simulink model "HVDCMMCInterconnection"  (R2023b)
settings: Solver=FixedStepDiscrete  StartTime=0.0  StopTime=10  FixedStep=Ts_Power  RelTol=1e-4
PreLoadFcn:
  | HVDCMMCInterconnectionParam
StartFcn:
  | tic
StopFcn:
  | toc
values from neighbouring files (symbols this model uses):
  C_PM = 1.758e-3    (= 0.001758)    [HVDCMMCInterconnectionParam.m]
  Cg = 50e-9    (= 5e-08)    [HVDCMMCInterconnectionParam.m]
  D_R = 0.001    [HVDCMMCInterconnectionParam.m]
  D_Rs = 1e8    (= 100000000)    [HVDCMMCInterconnectionParam.m]
  D_Vf = 0    [HVDCMMCInterconnectionParam.m]
  Fnom = 50    [HVDCMMCInterconnectionParam.m]
  HRM = 2    [HVDCMMCInterconnectionParam.m]
  Ki_Ireg = 6    [HVDCMMCInterconnectionParam.m]
  Ki_Preg = 1.0    (= 1)    [HVDCMMCInterconnectionParam.m]
  Ki_Qreg = 1.0    (= 1)    [HVDCMMCInterconnectionParam.m]
  Ki_VDCreg = 100    [HVDCMMCInterconnectionParam.m]
  Kp_Ireg = 0.6    [HVDCMMCInterconnectionParam.m]
  Kp_Preg = 0.5/3    (= 0.166666666667)    [HVDCMMCInterconnectionParam.m]
  Kp_Qreg = 0.5/3    (= 0.166666666667)    [HVDCMMCInterconnectionParam.m]
  Kp_VDCreg = 4    [HVDCMMCInterconnectionParam.m]
  L_cable = 15e-3    (= 0.015)    [HVDCMMCInterconnectionParam.m]
  Larm = Larm_pu*(Zb_ac/(2*pi*Fnom))    [HVDCMMCInterconnectionParam.m]
  Lff = Larm_pu/2    (= 0.075)    [HVDCMMCInterconnectionParam.m]
  Limits_Ireg = [ 2.0  -2.0]    [HVDCMMCInterconnectionParam.m]
  Limits_Preg = [ 1.2, 0.8 ]    [HVDCMMCInterconnectionParam.m]
  Limits_Qreg = [ 0.25, -0.25 ]    [HVDCMMCInterconnectionParam.m]
  Limits_VDCreg = [ 2.0  -2.0]    [HVDCMMCInterconnectionParam.m]
  Lxfo = 0.12    [HVDCMMCInterconnectionParam.m]
  Nb_PM = 36    [HVDCMMCInterconnectionParam.m]
  Pnom = 1000e6    (= 1000000000)    [HVDCMMCInterconnectionParam.m]
  R_cable = 0.5    [HVDCMMCInterconnectionParam.m]
  R_startup = 400    [HVDCMMCInterconnectionParam.m]
  Rarm = Rarm_pu*Zb_ac    [HVDCMMCInterconnectionParam.m]
  Rff = Rarm_pu/2    (= 0.00075)    [HVDCMMCInterconnectionParam.m]
  Rg = 100    [HVDCMMCInterconnectionParam.m]
  Rxfo = 0.003    [HVDCMMCInterconnectionParam.m]
  Slope_Pref = 0.5    [HVDCMMCInterconnectionParam.m]
  Slope_Qref = 0.5    [HVDCMMCInterconnectionParam.m]
  Slope_Vdc_ref = Vnom_dc/5    (= 128000)    [HVDCMMCInterconnectionParam.m]
  Tbrk1_On = 0.1    [HVDCMMCInterconnectionParam.m]
  Tbrk2_On = 1.0    (= 1)    [HVDCMMCInterconnectionParam.m]
  Tdeblock = 1.5    [HVDCMMCInterconnectionParam.m]
  Tfault = 9999    [HVDCMMCInterconnectionParam.m]
  Ton_Converter2 = 4    [HVDCMMCInterconnectionParam.m]
  Ton_PQreg = 4    [HVDCMMCInterconnectionParam.m]
  Ton_VDCreg = 1.5    [HVDCMMCInterconnectionParam.m]
  Ts = Ts_Control    (= 4e-05)    [HVDCMMCInterconnectionParam.m]    (also in power_circ2ss_sps_calc.m = 1e-06)
  Ts_Control = 40e-6    (= 4e-05)    [HVDCMMCInterconnectionParam.m]
  Ts_Power = 20e-6    (= 2e-05)    [HVDCMMCInterconnectionParam.m]
  Vb_ac = sqrt(2/3)*Vnom_sec    [HVDCMMCInterconnectionParam.m]
  Vb_dc = Vnom_dc    (= 640000)    [HVDCMMCInterconnectionParam.m]
  Vc0_PM = 0    [HVDCMMCInterconnectionParam.m]
  Vnom_dc = 640e3    (= 640000)    [HVDCMMCInterconnectionParam.m]
  Vnom_prim = 400e3    (= 400000)    [HVDCMMCInterconnectionParam.m]
  Vnom_sec = 333e3    (= 333000)    [HVDCMMCInterconnectionParam.m]
  w = 2*pi*Fnom    (= 314.159265359)    [HVDCMMCInterconnectionParam.m]
undefined symbols (not defined in the file or in its folder): ACDC, ACDC3, DiscIntNeverNeededParam, gcbh, Pcc, S, sps_AC, sps_rtmsupport
libraries: simulink x61, spsControlledVoltageSourceLib x56, spsCurrentMeasurementLib x56, spsDiodeLib x40, spsSeriesRLCBranchLib x32, spsVoltageMeasurementLib x20, powerlib_extras x9, spsHalfBridgeMMCmodel x8, spsGroundLib x7, spsSecondOrderFilterLib x6, spsabctodq0Lib x6, spsMeanLib x3
(part 2 of 11)

== system HVDCMMCInterconnection/3ph SM1 ==
  Uref_An : Inport
  An_Ipos : Inport  Port=2
  An_Icap : Inport  Port=3
  Demux : Demux  Outputs=2
  Demux2 : Demux  Outputs=2
  Discrete-Time Integrator1 : DiscreteIntegrator  IntegratorMethod=Integration: Trapezoidal  gainval=1  SampleTime=Ts_Power  UpperSaturationLimit=5000  LowerSaturationLimit=500  ICPrevOutput=DiscIntNeverNeededParam  ICPrevScaledInput=DiscIntNeverNeededParam
  Gain1 : Gain  Gain=Nb_PM
  Gain4 : Gain  Gain=1/(C_PM*Nb_PM)
  Gain5 : Gain  Gain=2
  Mux1 : Mux  Inputs=2
  Mux2 : Mux  Inputs=2
  Product3 : Product
  Product4 : Product
  Product7 : Product
  Sum3 : Sum  Inputs=1  InputSameDT=on  SaturateOnIntegerOverflow=on  OutDataTypeStr=Inherit: Same as first input
  Sum4 : Sum  Inputs=+-  InputSameDT=on  SaturateOnIntegerOverflow=on  OutDataTypeStr=Inherit: Same as first input
  Unit Delay5 : UnitDelay  SampleTime=Ts_Power  HasFrameUpgradeWarning=on
  Unit Delay6 : UnitDelay  SampleTime=Ts_Power  HasFrameUpgradeWarning=on
  Unit Delay7 : UnitDelay  SampleTime=Ts_Power  HasFrameUpgradeWarning=on
  An_Vbl : Outport
  An_Vin : Outport  Port=2
  wires:
  Gain5/1 -> Sum4/1
  Gain1/1 -> Demux2/1, Product3/1
  Mux2/1 -> Demux/1
  Demux/1 -> An_Vin/1
  Uref_An/1 -> Gain1/1
  Gain4/1 -> Discrete-Time Integrator1/1
  Mux1/1 -> Unit Delay7/1
  Demux2/2 -> Product7/1
  Unit Delay6/1 -> Gain5/1, Unit Delay5/1
  An_Icap/1 -> Mux1/2
  Demux2/1 -> Product4/1
  Discrete-Time Integrator1/1 -> Unit Delay6/1
  Sum4/1 -> Product7/2, Product4/2  "Vc"
  Unit Delay5/1 -> Sum4/2
  Sum3/1 -> Gain4/1
  Product3/1 -> Sum3/1
  Product4/1 -> Mux2/1  "Vin"
  Demux/2 -> An_Vbl/1
  Product7/1 -> Mux2/2  "Vbl"
  Unit Delay7/1 -> Product3/2
  An_Ipos/1 -> Mux1/1

== system HVDCMMCInterconnection/3ph SM10 ==
  Uref_An : Inport
  An_Ipos : Inport  Port=2
  An_Icap : Inport  Port=3
  Demux : Demux  Outputs=2
  Demux2 : Demux  Outputs=2
  Discrete-Time Integrator1 : DiscreteIntegrator  IntegratorMethod=Integration: Trapezoidal  gainval=1  SampleTime=Ts_Power  UpperSaturationLimit=5000  LowerSaturationLimit=500  ICPrevOutput=DiscIntNeverNeededParam  ICPrevScaledInput=DiscIntNeverNeededParam
  Gain1 : Gain  Gain=Nb_PM
  Gain4 : Gain  Gain=1/(C_PM*Nb_PM)
  Gain5 : Gain  Gain=2
  Mux1 : Mux  Inputs=2
  Mux2 : Mux  Inputs=2
  Product3 : Product
  Product4 : Product
  Product7 : Product
  Sum3 : Sum  Inputs=1  InputSameDT=on  SaturateOnIntegerOverflow=on  OutDataTypeStr=Inherit: Same as first input
  Sum4 : Sum  Inputs=+-  InputSameDT=on  SaturateOnIntegerOverflow=on  OutDataTypeStr=Inherit: Same as first input
  Unit Delay5 : UnitDelay  SampleTime=Ts_Power  HasFrameUpgradeWarning=on
  Unit Delay6 : UnitDelay  SampleTime=Ts_Power  HasFrameUpgradeWarning=on
  Unit Delay7 : UnitDelay  SampleTime=Ts_Power  HasFrameUpgradeWarning=on
  An_Vbl : Outport
  An_Vin : Outport  Port=2
  wires:
  Gain5/1 -> Sum4/1
  Gain1/1 -> Demux2/1, Product3/1
  Mux2/1 -> Demux/1
  Demux/1 -> An_Vin/1
  Uref_An/1 -> Gain1/1
  Gain4/1 -> Discrete-Time Integrator1/1
  Mux1/1 -> Unit Delay7/1
  Demux2/2 -> Product7/1
  Unit Delay6/1 -> Gain5/1, Unit Delay5/1
  An_Icap/1 -> Mux1/2
  Demux2/1 -> Product4/1
  Discrete-Time Integrator1/1 -> Unit Delay6/1
  Sum4/1 -> Product7/2, Product4/2  "Vc"
  Unit Delay5/1 -> Sum4/2
  Sum3/1 -> Gain4/1
  Product3/1 -> Sum3/1
  Product4/1 -> Mux2/1  "Vin"
  Demux/2 -> An_Vbl/1
  Product7/1 -> Mux2/2  "Vbl"
  Unit Delay7/1 -> Product3/2
  An_Ipos/1 -> Mux1/1

== system HVDCMMCInterconnection/3ph SM11 ==
  Uref_An : Inport
  An_Ipos : Inport  Port=2
  An_Icap : Inport  Port=3
  Demux : Demux  Outputs=2
  Demux2 : Demux  Outputs=2
  Discrete-Time Integrator1 : DiscreteIntegrator  IntegratorMethod=Integration: Trapezoidal  gainval=1  SampleTime=Ts_Power  UpperSaturationLimit=5000  LowerSaturationLimit=500  ICPrevOutput=DiscIntNeverNeededParam  ICPrevScaledInput=DiscIntNeverNeededParam
  Gain1 : Gain  Gain=Nb_PM
  Gain4 : Gain  Gain=1/(C_PM*Nb_PM)
  Gain5 : Gain  Gain=2
  Mux1 : Mux  Inputs=2
  Mux2 : Mux  Inputs=2
  Product3 : Product
  Product4 : Product
  Product7 : Product
  Sum3 : Sum  Inputs=1  InputSameDT=on  SaturateOnIntegerOverflow=on  OutDataTypeStr=Inherit: Same as first input
  Sum4 : Sum  Inputs=+-  InputSameDT=on  SaturateOnIntegerOverflow=on  OutDataTypeStr=Inherit: Same as first input
  Unit Delay5 : UnitDelay  SampleTime=Ts_Power  HasFrameUpgradeWarning=on
  Unit Delay6 : UnitDelay  SampleTime=Ts_Power  HasFrameUpgradeWarning=on
  Unit Delay7 : UnitDelay  SampleTime=Ts_Power  HasFrameUpgradeWarning=on
  An_Vbl : Outport
  An_Vin : Outport  Port=2
  wires:
  Gain5/1 -> Sum4/1
  Gain1/1 -> Demux2/1, Product3/1
  Mux2/1 -> Demux/1
  Demux/1 -> An_Vin/1
  Uref_An/1 -> Gain1/1
  Gain4/1 -> Discrete-Time Integrator1/1
  Mux1/1 -> Unit Delay7/1
  Demux2/2 -> Product7/1
  Unit Delay6/1 -> Gain5/1, Unit Delay5/1
  An_Icap/1 -> Mux1/2
  Demux2/1 -> Product4/1
  Discrete-Time Integrator1/1 -> Unit Delay6/1
  Sum4/1 -> Product7/2, Product4/2  "Vc"
  Unit Delay5/1 -> Sum4/2
  Sum3/1 -> Gain4/1
  Product3/1 -> Sum3/1
  Product4/1 -> Mux2/1  "Vin"
  Demux/2 -> An_Vbl/1
  Product7/1 -> Mux2/2  "Vbl"
  Unit Delay7/1 -> Product3/2
  An_Ipos/1 -> Mux1/1

== system HVDCMMCInterconnection/3ph SM12 ==
  Uref_An : Inport
  An_Ipos : Inport  Port=2
  An_Icap : Inport  Port=3
  Demux : Demux  Outputs=2
  Demux2 : Demux  Outputs=2
  Discrete-Time Integrator1 : DiscreteIntegrator  IntegratorMethod=Integration: Trapezoidal  gainval=1  SampleTime=Ts_Power  UpperSaturationLimit=5000  LowerSaturationLimit=500  ICPrevOutput=DiscIntNeverNeededParam  ICPrevScaledInput=DiscIntNeverNeededParam
  Gain1 : Gain  Gain=Nb_PM
  Gain4 : Gain  Gain=1/(C_PM*Nb_PM)
  Gain5 : Gain  Gain=2
  Mux1 : Mux  Inputs=2
  Mux2 : Mux  Inputs=2
  Product3 : Product
  Product4 : Product
  Product7 : Product
  Sum3 : Sum  Inputs=1  InputSameDT=on  SaturateOnIntegerOverflow=on  OutDataTypeStr=Inherit: Same as first input
  Sum4 : Sum  Inputs=+-  InputSameDT=on  SaturateOnIntegerOverflow=on  OutDataTypeStr=Inherit: Same as first input
  Unit Delay5 : UnitDelay  SampleTime=Ts_Power  HasFrameUpgradeWarning=on
  Unit Delay6 : UnitDelay  SampleTime=Ts_Power  HasFrameUpgradeWarning=on
  Unit Delay7 : UnitDelay  SampleTime=Ts_Power  HasFrameUpgradeWarning=on
  An_Vbl : Outport
  An_Vin : Outport  Port=2
  wires:
  Gain5/1 -> Sum4/1
  Gain1/1 -> Demux2/1, Product3/1
  Mux2/1 -> Demux/1
  Demux/1 -> An_Vin/1
  Uref_An/1 -> Gain1/1
  Gain4/1 -> Discrete-Time Integrator1/1
  Mux1/1 -> Unit Delay7/1
  Demux2/2 -> Product7/1
  Unit Delay6/1 -> Gain5/1, Unit Delay5/1
  An_Icap/1 -> Mux1/2
  Demux2/1 -> Product4/1
  Discrete-Time Integrator1/1 -> Unit Delay6/1
  Sum4/1 -> Product7/2, Product4/2  "Vc"
  Unit Delay5/1 -> Sum4/2
  Sum3/1 -> Gain4/1
  Product3/1 -> Sum3/1
  Product4/1 -> Mux2/1  "Vin"
  Demux/2 -> An_Vbl/1
  Product7/1 -> Mux2/2  "Vbl"
  Unit Delay7/1 -> Product3/2
  An_Ipos/1 -> Mux1/1

== system HVDCMMCInterconnection/3ph SM13 ==
  Uref_An : Inport
  An_Ipos : Inport  Port=2
  An_Icap : Inport  Port=3
  Demux : Demux  Outputs=2
  Demux2 : Demux  Outputs=2
  Discrete-Time Integrator1 : DiscreteIntegrator  IntegratorMethod=Integration: Trapezoidal  gainval=1  SampleTime=Ts_Power  UpperSaturationLimit=5000  LowerSaturationLimit=500  ICPrevOutput=DiscIntNeverNeededParam  ICPrevScaledInput=DiscIntNeverNeededParam
  Gain1 : Gain  Gain=Nb_PM
  Gain4 : Gain  Gain=1/(C_PM*Nb_PM)
  Gain5 : Gain  Gain=2
  Mux1 : Mux  Inputs=2
  Mux2 : Mux  Inputs=2
  Product3 : Product
  Product4 : Product
  Product7 : Product
  Sum3 : Sum  Inputs=1  InputSameDT=on  SaturateOnIntegerOverflow=on  OutDataTypeStr=Inherit: Same as first input
  Sum4 : Sum  Inputs=+-  InputSameDT=on  SaturateOnIntegerOverflow=on  OutDataTypeStr=Inherit: Same as first input
  Unit Delay5 : UnitDelay  SampleTime=Ts_Power  HasFrameUpgradeWarning=on
  Unit Delay6 : UnitDelay  SampleTime=Ts_Power  HasFrameUpgradeWarning=on
  Unit Delay7 : UnitDelay  SampleTime=Ts_Power  HasFrameUpgradeWarning=on
  An_Vbl : Outport
  An_Vin : Outport  Port=2
  wires:
  Gain5/1 -> Sum4/1
  Gain1/1 -> Demux2/1, Product3/1
  Mux2/1 -> Demux/1
  Demux/1 -> An_Vin/1
  Uref_An/1 -> Gain1/1
  Gain4/1 -> Discrete-Time Integrator1/1
  Mux1/1 -> Unit Delay7/1
  Demux2/2 -> Product7/1
  Unit Delay6/1 -> Gain5/1, Unit Delay5/1
  An_Icap/1 -> Mux1/2
  Demux2/1 -> Product4/1
  Discrete-Time Integrator1/1 -> Unit Delay6/1
  Sum4/1 -> Product7/2, Product4/2  "Vc"
  Unit Delay5/1 -> Sum4/2
  Sum3/1 -> Gain4/1
  Product3/1 -> Sum3/1
  Product4/1 -> Mux2/1  "Vin"
  Demux/2 -> An_Vbl/1
  Product7/1 -> Mux2/2  "Vbl"
  Unit Delay7/1 -> Product3/2
  An_Ipos/1 -> Mux1/1

== system HVDCMMCInterconnection/3ph SM14 ==
  Uref_An : Inport
  An_Ipos : Inport  Port=2
  An_Icap : Inport  Port=3
  Demux : Demux  Outputs=2
  Demux2 : Demux  Outputs=2
  Discrete-Time Integrator1 : DiscreteIntegrator  IntegratorMethod=Integration: Trapezoidal  gainval=1  SampleTime=Ts_Power  UpperSaturationLimit=5000  LowerSaturationLimit=500  ICPrevOutput=DiscIntNeverNeededParam  ICPrevScaledInput=DiscIntNeverNeededParam
  Gain1 : Gain  Gain=Nb_PM
  Gain4 : Gain  Gain=1/(C_PM*Nb_PM)
  Gain5 : Gain  Gain=2
  Mux1 : Mux  Inputs=2
  Mux2 : Mux  Inputs=2
  Product3 : Product
  Product4 : Product
  Product7 : Product
  Sum3 : Sum  Inputs=1  InputSameDT=on  SaturateOnIntegerOverflow=on  OutDataTypeStr=Inherit: Same as first input
  Sum4 : Sum  Inputs=+-  InputSameDT=on  SaturateOnIntegerOverflow=on  OutDataTypeStr=Inherit: Same as first input
  Unit Delay5 : UnitDelay  SampleTime=Ts_Power  HasFrameUpgradeWarning=on
  Unit Delay6 : UnitDelay  SampleTime=Ts_Power  HasFrameUpgradeWarning=on
  Unit Delay7 : UnitDelay  SampleTime=Ts_Power  HasFrameUpgradeWarning=on
  An_Vbl : Outport
  An_Vin : Outport  Port=2
  wires:
  Gain5/1 -> Sum4/1
  Gain1/1 -> Demux2/1, Product3/1
  Mux2/1 -> Demux/1
  Demux/1 -> An_Vin/1
  Uref_An/1 -> Gain1/1
  Gain4/1 -> Discrete-Time Integrator1/1
  Mux1/1 -> Unit Delay7/1
  Demux2/2 -> Product7/1
  Unit Delay6/1 -> Gain5/1, Unit Delay5/1
  An_Icap/1 -> Mux1/2
  Demux2/1 -> Product4/1
  Discrete-Time Integrator1/1 -> Unit Delay6/1
  Sum4/1 -> Product7/2, Product4/2  "Vc"
  Unit Delay5/1 -> Sum4/2
  Sum3/1 -> Gain4/1
  Product3/1 -> Sum3/1
  Product4/1 -> Mux2/1  "Vin"
  Demux/2 -> An_Vbl/1
  Product7/1 -> Mux2/2  "Vbl"
  Unit Delay7/1 -> Product3/2
  An_Ipos/1 -> Mux1/1

== system HVDCMMCInterconnection/3ph SM2 ==
  Uref_Ap : Inport
  Ap_Ipos : Inport  Port=2
  Ap_Icap : Inport  Port=3
  Demux1 : Demux  Outputs=2
  Demux3 : Demux  Outputs=2
  Discrete-Time Integrator2 : DiscreteIntegrator  IntegratorMethod=Integration: Trapezoidal  gainval=1  SampleTime=Ts_Power  UpperSaturationLimit=5000  LowerSaturationLimit=500  ICPrevOutput=DiscIntNeverNeededParam  ICPrevScaledInput=DiscIntNeverNeededParam
  Gain2 : Gain  Gain=Nb_PM
  Gain3 : Gain  Gain=1/(C_PM*Nb_PM)
  Gain6 : Gain  Gain=2
  Mux3 : Mux  Inputs=2
  Mux4 : Mux  Inputs=2
  Product1 : Product
  Product2 : Product
  Product5 : Product
  Sum1 : Sum  Inputs=1  InputSameDT=on  SaturateOnIntegerOverflow=on  OutDataTypeStr=Inherit: Same as first input
  Sum2 : Sum  Inputs=+-  InputSameDT=on  SaturateOnIntegerOverflow=on  OutDataTypeStr=Inherit: Same as first input
  Unit Delay1 : UnitDelay  SampleTime=Ts_Power  HasFrameUpgradeWarning=on
  Unit Delay2 : UnitDelay  SampleTime=Ts_Power  HasFrameUpgradeWarning=on
  Unit Delay3 : UnitDelay  SampleTime=Ts_Power  HasFrameUpgradeWarning=on
  Ap_Vbl : Outport
  Ap_Vin : Outport  Port=2
  wires:
  Demux1/2 -> Ap_Vbl/1
  Ap_Ipos/1 -> Mux3/1
  Unit Delay3/1 -> Product1/2
  Product1/1 -> Sum1/1
  Sum1/1 -> Gain3/1
  Unit Delay1/1 -> Sum2/2
  Sum2/1 -> Product5/2, Product2/2  "Vc"
  Uref_Ap/1 -> Gain2/1
  Unit Delay2/1 -> Gain6/1, Unit Delay1/1
  Mux3/1 -> Unit Delay3/1
  Demux3/2 -> Product5/1
  Gain3/1 -> Discrete-Time Integrator2/1
  Gain2/1 -> Demux3/1, Product1/1
  Demux3/1 -> Product2/1
  Demux1/1 -> Ap_Vin/1
  Mux4/1 -> Demux1/1
  Product2/1 -> Mux4/1  "Vin"
  Discrete-Time Integrator2/1 -> Unit Delay2/1
  Ap_Icap/1 -> Mux3/2
  Gain6/1 -> Sum2/1
  Product5/1 -> Mux4/2  "Vbl"

== system HVDCMMCInterconnection/3ph SM3 ==
  Uref_An : Inport
  An_Ipos : Inport  Port=2
  An_Icap : Inport  Port=3
  Demux : Demux  Outputs=2
  Demux2 : Demux  Outputs=2
  Discrete-Time Integrator1 : DiscreteIntegrator  IntegratorMethod=Integration: Trapezoidal  gainval=1  SampleTime=Ts_Power  UpperSaturationLimit=5000  LowerSaturationLimit=500  ICPrevOutput=DiscIntNeverNeededParam  ICPrevScaledInput=DiscIntNeverNeededParam
  Gain1 : Gain  Gain=Nb_PM
  Gain4 : Gain  Gain=1/(C_PM*Nb_PM)
  Gain5 : Gain  Gain=2
  Mux1 : Mux  Inputs=2
  Mux2 : Mux  Inputs=2
  Product3 : Product
  Product4 : Product
  Product7 : Product
  Sum3 : Sum  Inputs=1  InputSameDT=on  SaturateOnIntegerOverflow=on  OutDataTypeStr=Inherit: Same as first input
  Sum4 : Sum  Inputs=+-  InputSameDT=on  SaturateOnIntegerOverflow=on  OutDataTypeStr=Inherit: Same as first input
  Unit Delay5 : UnitDelay  SampleTime=Ts_Power  HasFrameUpgradeWarning=on
  Unit Delay6 : UnitDelay  SampleTime=Ts_Power  HasFrameUpgradeWarning=on
  Unit Delay7 : UnitDelay  SampleTime=Ts_Power  HasFrameUpgradeWarning=on
  An_Vbl : Outport
  An_Vin : Outport  Port=2
  wires:
  Gain5/1 -> Sum4/1
  Gain1/1 -> Demux2/1, Product3/1
  Mux2/1 -> Demux/1
  Demux/1 -> An_Vin/1
  Uref_An/1 -> Gain1/1
  Gain4/1 -> Discrete-Time Integrator1/1
  Mux1/1 -> Unit Delay7/1
  Demux2/2 -> Product7/1
  Unit Delay6/1 -> Gain5/1, Unit Delay5/1
  An_Icap/1 -> Mux1/2
  Demux2/1 -> Product4/1
  Discrete-Time Integrator1/1 -> Unit Delay6/1
  Sum4/1 -> Product7/2, Product4/2  "Vc"
  Unit Delay5/1 -> Sum4/2
  Sum3/1 -> Gain4/1
  Product3/1 -> Sum3/1
  Product4/1 -> Mux2/1  "Vin"
  Demux/2 -> An_Vbl/1
  Product7/1 -> Mux2/2  "Vbl"
  Unit Delay7/1 -> Product3/2
  An_Ipos/1 -> Mux1/1

== system HVDCMMCInterconnection/3ph SM4 ==
  Uref_An : Inport
  An_Ipos : Inport  Port=2
  An_Icap : Inport  Port=3
  Demux : Demux  Outputs=2
  Demux2 : Demux  Outputs=2
  Discrete-Time Integrator1 : DiscreteIntegrator  IntegratorMethod=Integration: Trapezoidal  gainval=1  SampleTime=Ts_Power  UpperSaturationLimit=5000  LowerSaturationLimit=500  ICPrevOutput=DiscIntNeverNeededParam  ICPrevScaledInput=DiscIntNeverNeededParam
  Gain1 : Gain  Gain=Nb_PM
  Gain4 : Gain  Gain=1/(C_PM*Nb_PM)
  Gain5 : Gain  Gain=2
  Mux1 : Mux  Inputs=2
  Mux2 : Mux  Inputs=2
  Product3 : Product
  Product4 : Product
  Product7 : Product
  Sum3 : Sum  Inputs=1  InputSameDT=on  SaturateOnIntegerOverflow=on  OutDataTypeStr=Inherit: Same as first input
  Sum4 : Sum  Inputs=+-  InputSameDT=on  SaturateOnIntegerOverflow=on  OutDataTypeStr=Inherit: Same as first input
  Unit Delay5 : UnitDelay  SampleTime=Ts_Power  HasFrameUpgradeWarning=on
  Unit Delay6 : UnitDelay  SampleTime=Ts_Power  HasFrameUpgradeWarning=on
  Unit Delay7 : UnitDelay  SampleTime=Ts_Power  HasFrameUpgradeWarning=on
  An_Vbl : Outport
  An_Vin : Outport  Port=2
  wires:
  Gain5/1 -> Sum4/1
  Gain1/1 -> Demux2/1, Product3/1
  Mux2/1 -> Demux/1
  Demux/1 -> An_Vin/1
  Uref_An/1 -> Gain1/1
  Gain4/1 -> Discrete-Time Integrator1/1
  Mux1/1 -> Unit Delay7/1
  Demux2/2 -> Product7/1
  Unit Delay6/1 -> Gain5/1, Unit Delay5/1
  An_Icap/1 -> Mux1/2
  Demux2/1 -> Product4/1
  Discrete-Time Integrator1/1 -> Unit Delay6/1
  Sum4/1 -> Product7/2, Product4/2  "Vc"
  Unit Delay5/1 -> Sum4/2
  Sum3/1 -> Gain4/1
  Product3/1 -> Sum3/1
  Product4/1 -> Mux2/1  "Vin"
  Demux/2 -> An_Vbl/1
  Product7/1 -> Mux2/2  "Vbl"
  Unit Delay7/1 -> Product3/2
  An_Ipos/1 -> Mux1/1

== system HVDCMMCInterconnection/3ph SM5 ==
  Uref_An : Inport
  An_Ipos : Inport  Port=2
  An_Icap : Inport  Port=3
  Demux : Demux  Outputs=2
  Demux2 : Demux  Outputs=2
  Discrete-Time Integrator1 : DiscreteIntegrator  IntegratorMethod=Integration: Trapezoidal  gainval=1  SampleTime=Ts_Power  UpperSaturationLimit=5000  LowerSaturationLimit=500  ICPrevOutput=DiscIntNeverNeededParam  ICPrevScaledInput=DiscIntNeverNeededParam
  Gain1 : Gain  Gain=Nb_PM
  Gain4 : Gain  Gain=1/(C_PM*Nb_PM)
  Gain5 : Gain  Gain=2
  Mux1 : Mux  Inputs=2
  Mux2 : Mux  Inputs=2
  Product3 : Product
  Product4 : Product
  Product7 : Product
  Sum3 : Sum  Inputs=1  InputSameDT=on  SaturateOnIntegerOverflow=on  OutDataTypeStr=Inherit: Same as first input
  Sum4 : Sum  Inputs=+-  InputSameDT=on  SaturateOnIntegerOverflow=on  OutDataTypeStr=Inherit: Same as first input
  Unit Delay5 : UnitDelay  SampleTime=Ts_Power  HasFrameUpgradeWarning=on
  Unit Delay6 : UnitDelay  SampleTime=Ts_Power  HasFrameUpgradeWarning=on
  Unit Delay7 : UnitDelay  SampleTime=Ts_Power  HasFrameUpgradeWarning=on
  An_Vbl : Outport
  An_Vin : Outport  Port=2
  wires:
  Gain5/1 -> Sum4/1
  Gain1/1 -> Demux2/1, Product3/1
  Mux2/1 -> Demux/1
  Demux/1 -> An_Vin/1
  Uref_An/1 -> Gain1/1
  Gain4/1 -> Discrete-Time Integrator1/1
  Mux1/1 -> Unit Delay7/1
  Demux2/2 -> Product7/1
  Unit Delay6/1 -> Gain5/1, Unit Delay5/1
  An_Icap/1 -> Mux1/2
  Demux2/1 -> Product4/1
  Discrete-Time Integrator1/1 -> Unit Delay6/1
  Sum4/1 -> Product7/2, Product4/2  "Vc"
  Unit Delay5/1 -> Sum4/2
  Sum3/1 -> Gain4/1
  Product3/1 -> Sum3/1
  Product4/1 -> Mux2/1  "Vin"
  Demux/2 -> An_Vbl/1
  Product7/1 -> Mux2/2  "Vbl"
  Unit Delay7/1 -> Product3/2
  An_Ipos/1 -> Mux1/1

== system HVDCMMCInterconnection/3ph SM6 ==
  Uref_An : Inport
  An_Ipos : Inport  Port=2
  An_Icap : Inport  Port=3
  Demux : Demux  Outputs=2
  Demux2 : Demux  Outputs=2
  Discrete-Time Integrator1 : DiscreteIntegrator  IntegratorMethod=Integration: Trapezoidal  gainval=1  SampleTime=Ts_Power  UpperSaturationLimit=5000  LowerSaturationLimit=500  ICPrevOutput=DiscIntNeverNeededParam  ICPrevScaledInput=DiscIntNeverNeededParam
  Gain1 : Gain  Gain=Nb_PM
  Gain4 : Gain  Gain=1/(C_PM*Nb_PM)
  Gain5 : Gain  Gain=2
  Mux1 : Mux  Inputs=2
  Mux2 : Mux  Inputs=2
  Product3 : Product
  Product4 : Product
  Product7 : Product
  Sum3 : Sum  Inputs=1  InputSameDT=on  SaturateOnIntegerOverflow=on  OutDataTypeStr=Inherit: Same as first input
  Sum4 : Sum  Inputs=+-  InputSameDT=on  SaturateOnIntegerOverflow=on  OutDataTypeStr=Inherit: Same as first input
  Unit Delay5 : UnitDelay  SampleTime=Ts_Power  HasFrameUpgradeWarning=on
  Unit Delay6 : UnitDelay  SampleTime=Ts_Power  HasFrameUpgradeWarning=on
  Unit Delay7 : UnitDelay  SampleTime=Ts_Power  HasFrameUpgradeWarning=on
  An_Vbl : Outport
  An_Vin : Outport  Port=2
  wires:
  Gain5/1 -> Sum4/1
  Gain1/1 -> Demux2/1, Product3/1
  Mux2/1 -> Demux/1
  Demux/1 -> An_Vin/1
  Uref_An/1 -> Gain1/1
  Gain4/1 -> Discrete-Time Integrator1/1
  Mux1/1 -> Unit Delay7/1
  Demux2/2 -> Product7/1
  Unit Delay6/1 -> Gain5/1, Unit Delay5/1
  An_Icap/1 -> Mux1/2
  Demux2/1 -> Product4/1
  Discrete-Time Integrator1/1 -> Unit Delay6/1
  Sum4/1 -> Product7/2, Product4/2  "Vc"
  Unit Delay5/1 -> Sum4/2
  Sum3/1 -> Gain4/1
  Product3/1 -> Sum3/1
  Product4/1 -> Mux2/1  "Vin"
  Demux/2 -> An_Vbl/1
  Product7/1 -> Mux2/2  "Vbl"
  Unit Delay7/1 -> Product3/2
  An_Ipos/1 -> Mux1/1

== system HVDCMMCInterconnection/3ph SM7 ==
  Uref_An : Inport
  An_Ipos : Inport  Port=2
  An_Icap : Inport  Port=3
  Demux : Demux  Outputs=2
  Demux2 : Demux  Outputs=2
  Discrete-Time Integrator1 : DiscreteIntegrator  IntegratorMethod=Integration: Trapezoidal  gainval=1  SampleTime=Ts_Power  UpperSaturationLimit=5000  LowerSaturationLimit=500  ICPrevOutput=DiscIntNeverNeededParam  ICPrevScaledInput=DiscIntNeverNeededParam
  Gain1 : Gain  Gain=Nb_PM
  Gain4 : Gain  Gain=1/(C_PM*Nb_PM)
  Gain5 : Gain  Gain=2
  Mux1 : Mux  Inputs=2
  Mux2 : Mux  Inputs=2
  Product3 : Product
  Product4 : Product
  Product7 : Product
  Sum3 : Sum  Inputs=1  InputSameDT=on  SaturateOnIntegerOverflow=on  OutDataTypeStr=Inherit: Same as first input
  Sum4 : Sum  Inputs=+-  InputSameDT=on  SaturateOnIntegerOverflow=on  OutDataTypeStr=Inherit: Same as first input
  Unit Delay5 : UnitDelay  SampleTime=Ts_Power  HasFrameUpgradeWarning=on
  Unit Delay6 : UnitDelay  SampleTime=Ts_Power  HasFrameUpgradeWarning=on
  Unit Delay7 : UnitDelay  SampleTime=Ts_Power  HasFrameUpgradeWarning=on
  An_Vbl : Outport
  An_Vin : Outport  Port=2
  wires:
  Gain5/1 -> Sum4/1
  Gain1/1 -> Demux2/1, Product3/1
  Mux2/1 -> Demux/1
  Demux/1 -> An_Vin/1
  Uref_An/1 -> Gain1/1
  Gain4/1 -> Discrete-Time Integrator1/1
  Mux1/1 -> Unit Delay7/1
  Demux2/2 -> Product7/1
  Unit Delay6/1 -> Gain5/1, Unit Delay5/1
  An_Icap/1 -> Mux1/2
  Demux2/1 -> Product4/1
  Discrete-Time Integrator1/1 -> Unit Delay6/1
  Sum4/1 -> Product7/2, Product4/2  "Vc"
  Unit Delay5/1 -> Sum4/2
  Sum3/1 -> Gain4/1
  Product3/1 -> Sum3/1
  Product4/1 -> Mux2/1  "Vin"
  Demux/2 -> An_Vbl/1
  Product7/1 -> Mux2/2  "Vbl"
  Unit Delay7/1 -> Product3/2
  An_Ipos/1 -> Mux1/1

== system HVDCMMCInterconnection/3ph SM8 ==
  Uref_An : Inport
  An_Ipos : Inport  Port=2
  An_Icap : Inport  Port=3
  Demux : Demux  Outputs=2
  Demux2 : Demux  Outputs=2
  Discrete-Time Integrator1 : DiscreteIntegrator  IntegratorMethod=Integration: Trapezoidal  gainval=1  SampleTime=Ts_Power  UpperSaturationLimit=5000  LowerSaturationLimit=500  ICPrevOutput=DiscIntNeverNeededParam  ICPrevScaledInput=DiscIntNeverNeededParam
  Gain1 : Gain  Gain=Nb_PM
  Gain4 : Gain  Gain=1/(C_PM*Nb_PM)
  Gain5 : Gain  Gain=2
  Mux1 : Mux  Inputs=2
  Mux2 : Mux  Inputs=2
  Product3 : Product
  Product4 : Product
  Product7 : Product
  Sum3 : Sum  Inputs=1  InputSameDT=on  SaturateOnIntegerOverflow=on  OutDataTypeStr=Inherit: Same as first input
  Sum4 : Sum  Inputs=+-  InputSameDT=on  SaturateOnIntegerOverflow=on  OutDataTypeStr=Inherit: Same as first input
  Unit Delay5 : UnitDelay  SampleTime=Ts_Power  HasFrameUpgradeWarning=on
  Unit Delay6 : UnitDelay  SampleTime=Ts_Power  HasFrameUpgradeWarning=on
  Unit Delay7 : UnitDelay  SampleTime=Ts_Power  HasFrameUpgradeWarning=on
  An_Vbl : Outport
  An_Vin : Outport  Port=2
  wires:
  Gain5/1 -> Sum4/1
  Gain1/1 -> Demux2/1, Product3/1
  Mux2/1 -> Demux/1
  Demux/1 -> An_Vin/1
  Uref_An/1 -> Gain1/1
  Gain4/1 -> Discrete-Time Integrator1/1
  Mux1/1 -> Unit Delay7/1
  Demux2/2 -> Product7/1
  Unit Delay6/1 -> Gain5/1, Unit Delay5/1
  An_Icap/1 -> Mux1/2
  Demux2/1 -> Product4/1
  Discrete-Time Integrator1/1 -> Unit Delay6/1
  Sum4/1 -> Product7/2, Product4/2  "Vc"
  Unit Delay5/1 -> Sum4/2
  Sum3/1 -> Gain4/1
  Product3/1 -> Sum3/1
  Product4/1 -> Mux2/1  "Vin"
  Demux/2 -> An_Vbl/1
  Product7/1 -> Mux2/2  "Vbl"
  Unit Delay7/1 -> Product3/2
  An_Ipos/1 -> Mux1/1

== system HVDCMMCInterconnection/3ph SM9 ==
  Uref_An : Inport
  An_Ipos : Inport  Port=2
  An_Icap : Inport  Port=3
  Demux : Demux  Outputs=2
  Demux2 : Demux  Outputs=2
  Discrete-Time Integrator1 : DiscreteIntegrator  IntegratorMethod=Integration: Trapezoidal  gainval=1  SampleTime=Ts_Power  UpperSaturationLimit=5000  LowerSaturationLimit=500  ICPrevOutput=DiscIntNeverNeededParam  ICPrevScaledInput=DiscIntNeverNeededParam
  Gain1 : Gain  Gain=Nb_PM
  Gain4 : Gain  Gain=1/(C_PM*Nb_PM)
  Gain5 : Gain  Gain=2
  Mux1 : Mux  Inputs=2
  Mux2 : Mux  Inputs=2
  Product3 : Product
  Product4 : Product
  Product7 : Product
  Sum3 : Sum  Inputs=1  InputSameDT=on  SaturateOnIntegerOverflow=on  OutDataTypeStr=Inherit: Same as first input
  Sum4 : Sum  Inputs=+-  InputSameDT=on  SaturateOnIntegerOverflow=on  OutDataTypeStr=Inherit: Same as first input
  Unit Delay5 : UnitDelay  SampleTime=Ts_Power  HasFrameUpgradeWarning=on
  Unit Delay6 : UnitDelay  SampleTime=Ts_Power  HasFrameUpgradeWarning=on
  Unit Delay7 : UnitDelay  SampleTime=Ts_Power  HasFrameUpgradeWarning=on
  An_Vbl : Outport
  An_Vin : Outport  Port=2
  wires:
  Gain5/1 -> Sum4/1
  Gain1/1 -> Demux2/1, Product3/1
  Mux2/1 -> Demux/1
  Demux/1 -> An_Vin/1
  Uref_An/1 -> Gain1/1
  Gain4/1 -> Discrete-Time Integrator1/1
  Mux1/1 -> Unit Delay7/1
  Demux2/2 -> Product7/1
  Unit Delay6/1 -> Gain5/1, Unit Delay5/1
  An_Icap/1 -> Mux1/2
  Demux2/1 -> Product4/1
  Discrete-Time Integrator1/1 -> Unit Delay6/1
  Sum4/1 -> Product7/2, Product4/2  "Vc"
  Unit Delay5/1 -> Sum4/2
  Sum3/1 -> Gain4/1
  Product3/1 -> Sum3/1
  Product4/1 -> Mux2/1  "Vin"
  Demux/2 -> An_Vbl/1
  Product7/1 -> Mux2/2  "Vbl"
  Unit Delay7/1 -> Product3/2
  An_Ipos/1 -> Mux1/1

== system HVDCMMCInterconnection/BRK_CTRL ==
  UBrk1_EMT : Inport
  Brk_ON : Inport  Port=2
  Cast To Double{,1..3} (4 alike) : DataTypeConversion  OutDataTypeStr=double  SaturateOnIntegerOverflow=off  RndMeth=Floor
  Compare To Constant4 : simulink/Logic and Bit Operations/Compare To Constant  relop=>  const=0  OutDataTypeStr=boolean
  Gain : Gain  Gain=1/1e6
  Gain3 : Gain  Gain=1/0.01
  MUX2 : Subsystem
  NOT2 : Logic  Operator=NOT  IconShape=distinctive  AllPortsSameDT=off  OutDataTypeStr=boolean
  Product : Product
  Product1 : Product
  IBrk1_ss : Outport
  wires:
  Cast To Double1/1 -> Product/2
  Product1/1 -> MUX2/2(In2)
  UBrk1_EMT/1 -> Gain3/1, Gain/1
  Compare To Constant4/1 -> Cast To Double1/1, NOT2/1
  Product/1 -> MUX2/1(In1)
  Gain/1 -> Cast To Double3/1
  NOT2/1 -> Cast To Double2/1
  Cast To Double/1 -> Product/1
  Gain3/1 -> Cast To Double/1
  Cast To Double3/1 -> Product1/2
  Brk_ON/1 -> Compare To Constant4/1
  Cast To Double2/1 -> Product1/1
  MUX2/1(Out1) -> IBrk1_ss/1  "IBrk1_ss"

== system HVDCMMCInterconnection/BRK_CTRL1 ==
  UBrk1_EMT : Inport
  Brk_ON : Inport  Port=2
  Cast To Double{,1..3} (4 alike) : DataTypeConversion  OutDataTypeStr=double  SaturateOnIntegerOverflow=off  RndMeth=Floor
  Compare To Constant4 : simulink/Logic and Bit Operations/Compare To Constant  relop=>  const=0  OutDataTypeStr=boolean
  Gain : Gain  Gain=1/1e6
  Gain3 : Gain  Gain=1/0.01
  MUX2 : Subsystem
  NOT2 : Logic  Operator=NOT  IconShape=distinctive  AllPortsSameDT=off  OutDataTypeStr=boolean
  Product : Product
  Product1 : Product
  IBrk1_ss : Outport
  wires:
  Cast To Double1/1 -> Product/2
  Product1/1 -> MUX2/2(In2)
  UBrk1_EMT/1 -> Gain3/1, Gain/1
  Compare To Constant4/1 -> Cast To Double1/1, NOT2/1
  Product/1 -> MUX2/1(In1)
  Gain/1 -> Cast To Double3/1
  NOT2/1 -> Cast To Double2/1
  Cast To Double/1 -> Product/1
  Gain3/1 -> Cast To Double/1
  Cast To Double3/1 -> Product1/2
  Brk_ON/1 -> Compare To Constant4/1
  Cast To Double2/1 -> Product1/1
  MUX2/1(Out1) -> IBrk1_ss/1  "IBrk1_ss"

== system HVDCMMCInterconnection/Control ==
  PQreg_ON : Inport
  Vdc_ref : Inport  Port=2
  Qref : Inport  Port=3
  Vsec : Inport  Port=4
  Isec : Inport  Port=5
  Active Power Regulator (Preg) : Subsystem
  Bus Creator : BusCreator  Inputs=8
  Current Regulator (Ireg) : Subsystem
      settings: PortSchema="{\"entries\":[{\"content\":{\"sides\":[{\"content\":{\"connectorIds\":[\"In1\",\"In2\",\"In3\",\"In4\",\"In5\"]},\"type\":\"ConnectorPlacement.EquallySpacedRectSide\",\"uuid\":\"46fff04e-1450-479d-b460-437d90e99f23\"},{\"content\":{\"connectorIds\":[\"Out1\",\"Out2\",\"Out3\"],\"side\":\"RIGHT\"},\"type\":\"ConnectorPlacement.EquallySpacedRectSide\",\"uuid\":\"1fecc714-62d0-4152-98c9-212d930a5fef\"},{\"content\":{\"connectorIds\":[\"In6\"],\"side\":\"TOP\"},\"type\":\"ConnectorPlacement.EquallySpacedRectSide\",\"uuid\":\"861e6320-ec6e-4c2a-8449-e621a478dd1e\"}]},\"type\":\"ConnectorPlacement.EquallySpacedConnector\",\"uuid\":\"2e901dc7-e129-44fe-b6c0-1fa97996cfbd\"}],\"packageUris\":[\"http://schema.mathworks.com/mf0/Connector/R2020b\"],\"version\":\"1.0\"}"
  DC Voltage Regulator (VDCreg) : Subsystem
      settings: PortSchema="{\"entries\":[{\"content\":{\"sides\":[{\"content\":{\"connectorIds\":[\"In1\",\"In2\"]},\"type\":\"ConnectorPlacement.EquallySpacedRectSide\",\"uuid\":\"c20f24de-2933-46ae-a608-0dc6cbdc22c5\"},{\"content\":{\"connectorIds\":[\"Out1\"],\"side\":\"RIGHT\"},\"type\":\"ConnectorPlacement.EquallySpacedRectSide\",\"uuid\":\"78958689-3494-4241-b4e6-c71b7d261298\"},{\"content\":{\"connectorIds\":[\"In3\"],\"side\":\"TOP\"},\"type\":\"ConnectorPlacement.EquallySpacedRectSide\",\"uuid\":\"05cc66e2-c7d6-407f-b011-a28bc71811d6\"}]},\"type\":\"ConnectorPlacement.EquallySpacedConnector\",\"uuid\":\"0d848e7c-ac8e-4664-bac3-455723337427\"}],\"packageUris\":[\"http://schema.mathworks.com/mf0/Connector/R2020b\"],\"version\":\"1.0\"}"
  Demux1 : Demux  Outputs=2
  Demux3 : Demux  Outputs=2
  Mux : Mux  Inputs=2
  Mux1 : Mux  Inputs=2
  Mux2 : Mux  Inputs=2
  "PLL, Measurements and Transformation" : Subsystem
      settings: PortSchema="{\"entries\":[{\"content\":{\"sides\":[{\"content\":{\"connectorIds\":[\"In1\",\"In2\"]},\"type\":\"ConnectorPlacement.EquallySpacedRectSide\",\"uuid\":\"b10cca13-b0c2-430a-b17c-db71eb4f1a3c\"},{\"content\":{\"connectorIds\":[\"Out1\",\"Out2\",\"Out3\",\"Out4\"],\"side\":\"RIGHT\"},\"type\":\"ConnectorPlacement.EquallySpacedRectSide\",\"uuid\":\"355382eb-bc30-4f3c-94e5-48c8b9c2ecfd\"},{\"content\":{\"connectorIds\":[\"Out5\",\"Out6\"],\"side\":\"TOP\"},\"type\":\"ConnectorPlacement.EquallySpacedRectSide\",\"uuid\":\"77f94122-ff4d-41eb-b55d-9b38525f3ab4\"}]},\"type\":\"ConnectorPlacement.EquallySpacedConnector\",\"uuid\":\"46538cda-22c7-46a2-9cc9-63f6dc7214f2\"}],\"packageUris\":[\"http://schema.mathworks.com/mf0/Connector/R2020b\"],\"version\":\"1.0\"}"
  Rate Transition{,1..2,7} (4 alike) : RateTransition  OutPortSampleTime=Ts_Control
  Rate Transition11 : RateTransition  OutPortSampleTime=Ts_Power
  Rate Transition3 : RateTransition  OutPortSampleTime=Ts_Power
  Rate Transition4 : RateTransition  OutPortSampleTime=Ts_Power
  Reactive Power Regulator : Subsystem
      settings: PortSchema="{\"entries\":[{\"content\":{\"sides\":[{\"content\":{\"connectorIds\":[\"In1\",\"In2\"]},\"type\":\"ConnectorPlacement.EquallySpacedRectSide\",\"uuid\":\"eeeb811d-908b-486e-b0fa-0b5fd0d6695a\"},{\"content\":{\"connectorIds\":[\"Out1\"],\"side\":\"RIGHT\"},\"type\":\"ConnectorPlacement.EquallySpacedRectSide\",\"uuid\":\"28c9bf02-c5ab-433a-87a9-c17e67d0c029\"},{\"content\":{\"side\":\"TOP\"},\"type\":\"ConnectorPlacement.EquallySpacedRectSide\",\"uuid\":\"fdca837a-4079-4910-a6d7-edbb284eaa51\"},{\"content\":{\"connectorIds\":[\"In3\",\"In4\"],\"side\":\"BOTTOM\"},\"type\":\"ConnectorPlacement.EquallySpacedRectSide\",\"uuid\":\"d2fa5805-110b-4a78-bf6e-301fd334a724\"}]},\"type\":\"ConnectorPlacement.EquallySpacedConnector\",\"uuid\":\"cbc8ea8f-55f5-4ff6-b34f-d5812b415dcf\"}],\"packageUris\":[\"http://schema.mathworks.com/mf0/Connector/R2020b\"],\"version\":\"1.0\"}"
  Switch : Switch  Criteria=u2 ~= 0  SaturateOnIntegerOverflow=off  InputSameDT=off
  Uref : Outport
  Meas : Outport  Port=2
  m1_dq : Outport  Port=3
  wt : Outport  Port=4
  wires:
  Mux1/1 -> Bus Creator/7  "PrefPmeas"
  "PLL, Measurements and Transformation"/4(P) -> Mux1/2, Active Power Regulator (Preg)/1(Pmeas)
  DC Voltage Regulator (VDCreg)/1(Id_ref) -> Mux/1
  "PLL, Measurements and Transformation"/2(wt) -> Rate Transition4/1, Current Regulator (Ireg)/4(wt)
  Demux1/1 -> Bus Creator/3  "Id"
  Vsec/1 -> Rate Transition1/1
  "PLL, Measurements and Transformation"/6(VdVq) -> Reactive Power Regulator/4(VdVq_mes), Current Regulator (Ireg)/2(VdVq)
  Mux2/1 -> [QrefQmeas]
  Rate Transition11/1 -> Uref/1
  "PLL, Measurements and Transformation"/5(Q) -> Mux2/2, Reactive Power Regulator/3(Qmes)
  [Pref] -> Active Power Regulator (Preg)/2(Pref), Mux1/1
  Isec/1 -> Rate Transition2/1
  [PQreg_On] -> Active Power Regulator (Preg)/3(On)
  [QrefQmeas] -> Bus Creator/8  "QrefQmeas"
  Current Regulator (Ireg)/2(m) -> Rate Transition3/1, Rate Transition7/1
  Demux3/2 -> Bus Creator/2  "Iqref"
  Rate Transition7/1 -> Bus Creator/5  "m"
  [Vdc_ref_Preg] -> Switch/1
  Demux3/1 -> Bus Creator/1  "Idref"
  Mux/1 -> Demux3/1, Current Regulator (Ireg)/1(IdIq_ref)
  Switch/1 -> DC Voltage Regulator (VDCreg)/1(Vdc_ref)
  Current Regulator (Ireg)/3(PIdq) -> Bus Creator/6  "PIdq"
  [Vdc1] -> Rate Transition/1
  PQreg_ON/1 -> Reactive Power Regulator/1(On), Switch/2
  Rate Transition1/1 -> "PLL, Measurements and Transformation"/1(Vabc)
  "PLL, Measurements and Transformation"/1(Freq) -> Current Regulator (Ireg)/3(Freq)
  Vdc_ref/1 -> Switch/3
  Active Power Regulator (Preg)/1(Vdc_ref) -> [Vdc_ref_Preg]
  Rate Transition2/1 -> "PLL, Measurements and Transformation"/2(Iabc)
  Rate Transition/1 -> DC Voltage Regulator (VDCreg)/3(Vdc_meas), Current Regulator (Ireg)/6(Vdc)
  [VDCreg_On] -> DC Voltage Regulator (VDCreg)/2(On)
  Demux1/2 -> Bus Creator/4  "Iq"
  "PLL, Measurements and Transformation"/3(IdIq) -> Current Regulator (Ireg)/5(IdIq), Demux1/1
  Qref/1 -> Mux2/1, Reactive Power Regulator/2(Qref)
  Current Regulator (Ireg)/1(Uref_ABC) -> Rate Transition11/1
  Bus Creator/1 -> Meas/1
  Reactive Power Regulator/1(Iq_ref) -> Mux/2
  Rate Transition3/1 -> m1_dq/1
  Rate Transition4/1 -> wt/1

== system HVDCMMCInterconnection/Control1 ==
  PQreg_ON : Inport
  Vdc_ref : Inport  Port=2
  Qref : Inport  Port=3
  Vsec : Inport  Port=4
  Isec : Inport  Port=5
  Active Power Regulator (Preg) : Subsystem
  Bus Creator : BusCreator  Inputs=8
  Current Regulator (Ireg) : Subsystem
      settings: PortSchema="{\"entries\":[{\"content\":{\"sides\":[{\"content\":{\"connectorIds\":[\"In1\",\"In2\",\"In3\",\"In4\",\"In5\"]},\"type\":\"ConnectorPlacement.EquallySpacedRectSide\",\"uuid\":\"46fff04e-1450-479d-b460-437d90e99f23\"},{\"content\":{\"connectorIds\":[\"Out1\",\"Out2\",\"Out3\"],\"side\":\"RIGHT\"},\"type\":\"ConnectorPlacement.EquallySpacedRectSide\",\"uuid\":\"1fecc714-62d0-4152-98c9-212d930a5fef\"},{\"content\":{\"connectorIds\":[\"In6\"],\"side\":\"TOP\"},\"type\":\"ConnectorPlacement.EquallySpacedRectSide\",\"uuid\":\"861e6320-ec6e-4c2a-8449-e621a478dd1e\"}]},\"type\":\"ConnectorPlacement.EquallySpacedConnector\",\"uuid\":\"2e901dc7-e129-44fe-b6c0-1fa97996cfbd\"}],\"packageUris\":[\"http://schema.mathworks.com/mf0/Connector/R2020b\"],\"version\":\"1.0\"}"
  DC Voltage Regulator (VDCreg) : Subsystem
      settings: PortSchema="{\"entries\":[{\"content\":{\"sides\":[{\"content\":{\"connectorIds\":[\"In1\",\"In2\"]},\"type\":\"ConnectorPlacement.EquallySpacedRectSide\",\"uuid\":\"c20f24de-2933-46ae-a608-0dc6cbdc22c5\"},{\"content\":{\"connectorIds\":[\"Out1\"],\"side\":\"RIGHT\"},\"type\":\"ConnectorPlacement.EquallySpacedRectSide\",\"uuid\":\"78958689-3494-4241-b4e6-c71b7d261298\"},{\"content\":{\"connectorIds\":[\"In3\"],\"side\":\"TOP\"},\"type\":\"ConnectorPlacement.EquallySpacedRectSide\",\"uuid\":\"05cc66e2-c7d6-407f-b011-a28bc71811d6\"}]},\"type\":\"ConnectorPlacement.EquallySpacedConnector\",\"uuid\":\"0d848e7c-ac8e-4664-bac3-455723337427\"}],\"packageUris\":[\"http://schema.mathworks.com/mf0/Connector/R2020b\"],\"version\":\"1.0\"}"
  Demux1 : Demux  Outputs=2
  Demux3 : Demux  Outputs=2
  Mux : Mux  Inputs=2
  Mux1 : Mux  Inputs=2
  Mux2 : Mux  Inputs=2
  "PLL, Measurements and Transformation" : Subsystem
      settings: PortSchema="{\"entries\":[{\"content\":{\"sides\":[{\"content\":{\"connectorIds\":[\"In1\",\"In2\"]},\"type\":\"ConnectorPlacement.EquallySpacedRectSide\",\"uuid\":\"b10cca13-b0c2-430a-b17c-db71eb4f1a3c\"},{\"content\":{\"connectorIds\":[\"Out1\",\"Out2\",\"Out3\",\"Out4\"],\"side\":\"RIGHT\"},\"type\":\"ConnectorPlacement.EquallySpacedRectSide\",\"uuid\":\"355382eb-bc30-4f3c-94e5-48c8b9c2ecfd\"},{\"content\":{\"connectorIds\":[\"Out5\",\"Out6\"],\"side\":\"TOP\"},\"type\":\"ConnectorPlacement.EquallySpacedRectSide\",\"uuid\":\"77f94122-ff4d-41eb-b55d-9b38525f3ab4\"}]},\"type\":\"ConnectorPlacement.EquallySpacedConnector\",\"uuid\":\"46538cda-22c7-46a2-9cc9-63f6dc7214f2\"}],\"packageUris\":[\"http://schema.mathworks.com/mf0/Connector/R2020b\"],\"version\":\"1.0\"}"
  Rate Transition{,1..2,7} (4 alike) : RateTransition  OutPortSampleTime=Ts_Control
  Rate Transition11 : RateTransition  OutPortSampleTime=Ts_Power
  Rate Transition3 : RateTransition  OutPortSampleTime=Ts_Power
  Rate Transition4 : RateTransition  OutPortSampleTime=Ts_Power
  Reactive Power Regulator : Subsystem
      settings: PortSchema="{\"entries\":[{\"content\":{\"sides\":[{\"content\":{\"connectorIds\":[\"In1\",\"In2\"]},\"type\":\"ConnectorPlacement.EquallySpacedRectSide\",\"uuid\":\"eeeb811d-908b-486e-b0fa-0b5fd0d6695a\"},{\"content\":{\"connectorIds\":[\"Out1\"],\"side\":\"RIGHT\"},\"type\":\"ConnectorPlacement.EquallySpacedRectSide\",\"uuid\":\"28c9bf02-c5ab-433a-87a9-c17e67d0c029\"},{\"content\":{\"side\":\"TOP\"},\"type\":\"ConnectorPlacement.EquallySpacedRectSide\",\"uuid\":\"fdca837a-4079-4910-a6d7-edbb284eaa51\"},{\"content\":{\"connectorIds\":[\"In3\",\"In4\"],\"side\":\"BOTTOM\"},\"type\":\"ConnectorPlacement.EquallySpacedRectSide\",\"uuid\":\"d2fa5805-110b-4a78-bf6e-301fd334a724\"}]},\"type\":\"ConnectorPlacement.EquallySpacedConnector\",\"uuid\":\"cbc8ea8f-55f5-4ff6-b34f-d5812b415dcf\"}],\"packageUris\":[\"http://schema.mathworks.com/mf0/Connector/R2020b\"],\"version\":\"1.0\"}"
  Switch : Switch  Criteria=u2 ~= 0  SaturateOnIntegerOverflow=off  InputSameDT=off
  Uref : Outport
  Meas : Outport  Port=2
  m1_dq : Outport  Port=3
  wt : Outport  Port=4
  wires:
  Mux1/1 -> Bus Creator/7  "PrefPmeas"
  "PLL, Measurements and Transformation"/4(P) -> Mux1/2, Active Power Regulator (Preg)/1(Pmeas)
  DC Voltage Regulator (VDCreg)/1(Id_ref) -> Mux/1
  "PLL, Measurements and Transformation"/2(wt) -> Rate Transition4/1, Current Regulator (Ireg)/4(wt)
  Demux1/1 -> Bus Creator/3  "Id"
  Vsec/1 -> Rate Transition1/1
  "PLL, Measurements and Transformation"/6(VdVq) -> Reactive Power Regulator/4(VdVq_mes), Current Regulator (Ireg)/2(VdVq)
  Mux2/1 -> [QrefQmeas]
  Rate Transition11/1 -> Uref/1
  "PLL, Measurements and Transformation"/5(Q) -> Mux2/2, Reactive Power Regulator/3(Qmes)
  [Pref] -> Active Power Regulator (Preg)/2(Pref), Mux1/1
  Isec/1 -> Rate Transition2/1
  [PQreg_On] -> Active Power Regulator (Preg)/3(On)
  [QrefQmeas] -> Bus Creator/8  "QrefQmeas"
  Current Regulator (Ireg)/2(m) -> Rate Transition3/1, Rate Transition7/1
  Demux3/2 -> Bus Creator/2  "Iqref"
  Rate Transition7/1 -> Bus Creator/5  "m"
  [Vdc_ref_Preg] -> Switch/1
  Demux3/1 -> Bus Creator/1  "Idref"
  Mux/1 -> Demux3/1, Current Regulator (Ireg)/1(IdIq_ref)
  Switch/1 -> DC Voltage Regulator (VDCreg)/1(Vdc_ref)
  Current Regulator (Ireg)/3(PIdq) -> Bus Creator/6  "PIdq"
  [Vdc1] -> Rate Transition/1
  PQreg_ON/1 -> Reactive Power Regulator/1(On), Switch/2
  Rate Transition1/1 -> "PLL, Measurements and Transformation"/1(Vabc)
  "PLL, Measurements and Transformation"/1(Freq) -> Current Regulator (Ireg)/3(Freq)
  Vdc_ref/1 -> Switch/3
  Active Power Regulator (Preg)/1(Vdc_ref) -> [Vdc_ref_Preg]
  Rate Transition2/1 -> "PLL, Measurements and Transformation"/2(Iabc)
  Rate Transition/1 -> DC Voltage Regulator (VDCreg)/3(Vdc_meas), Current Regulator (Ireg)/6(Vdc)
  [VDCreg_On] -> DC Voltage Regulator (VDCreg)/2(On)
  Demux1/2 -> Bus Creator/4  "Iq"
  "PLL, Measurements and Transformation"/3(IdIq) -> Current Regulator (Ireg)/5(IdIq), Demux1/1
  Qref/1 -> Mux2/1, Reactive Power Regulator/2(Qref)
  Current Regulator (Ireg)/1(Uref_ABC) -> Rate Transition11/1
  Bus Creator/1 -> Meas/1
  Reactive Power Regulator/1(Iq_ref) -> Mux/2
  Rate Transition3/1 -> m1_dq/1
  Rate Transition4/1 -> wt/1

== system HVDCMMCInterconnection/Control2 ==
  PQreg_ON : Inport
  Vdc_ref : Inport  Port=2
  Qref : Inport  Port=3
  Vsec : Inport  Port=4
  Isec : Inport  Port=5
  Active Power Regulator (Preg) : Subsystem
  Bus Creator : BusCreator  Inputs=8
  Current Regulator (Ireg) : Subsystem
      settings: PortSchema="{\"entries\":[{\"content\":{\"sides\":[{\"content\":{\"connectorIds\":[\"In1\",\"In2\",\"In3\",\"In4\",\"In5\"]},\"type\":\"ConnectorPlacement.EquallySpacedRectSide\",\"uuid\":\"46fff04e-1450-479d-b460-437d90e99f23\"},{\"content\":{\"connectorIds\":[\"Out1\",\"Out2\",\"Out3\"],\"side\":\"RIGHT\"},\"type\":\"ConnectorPlacement.EquallySpacedRectSide\",\"uuid\":\"1fecc714-62d0-4152-98c9-212d930a5fef\"},{\"content\":{\"connectorIds\":[\"In6\"],\"side\":\"TOP\"},\"type\":\"ConnectorPlacement.EquallySpacedRectSide\",\"uuid\":\"861e6320-ec6e-4c2a-8449-e621a478dd1e\"}]},\"type\":\"ConnectorPlacement.EquallySpacedConnector\",\"uuid\":\"2e901dc7-e129-44fe-b6c0-1fa97996cfbd\"}],\"packageUris\":[\"http://schema.mathworks.com/mf0/Connector/R2020b\"],\"version\":\"1.0\"}"
  DC Voltage Regulator (VDCreg) : Subsystem
      settings: PortSchema="{\"entries\":[{\"content\":{\"sides\":[{\"content\":{\"connectorIds\":[\"In1\",\"In2\"]},\"type\":\"ConnectorPlacement.EquallySpacedRectSide\",\"uuid\":\"c20f24de-2933-46ae-a608-0dc6cbdc22c5\"},{\"content\":{\"connectorIds\":[\"Out1\"],\"side\":\"RIGHT\"},\"type\":\"ConnectorPlacement.EquallySpacedRectSide\",\"uuid\":\"78958689-3494-4241-b4e6-c71b7d261298\"},{\"content\":{\"connectorIds\":[\"In3\"],\"side\":\"TOP\"},\"type\":\"ConnectorPlacement.EquallySpacedRectSide\",\"uuid\":\"05cc66e2-c7d6-407f-b011-a28bc71811d6\"}]},\"type\":\"ConnectorPlacement.EquallySpacedConnector\",\"uuid\":\"0d848e7c-ac8e-4664-bac3-455723337427\"}],\"packageUris\":[\"http://schema.mathworks.com/mf0/Connector/R2020b\"],\"version\":\"1.0\"}"
  Demux1 : Demux  Outputs=2
  Demux3 : Demux  Outputs=2
  Mux : Mux  Inputs=2
  Mux1 : Mux  Inputs=2
  Mux2 : Mux  Inputs=2
  "PLL, Measurements and Transformation" : Subsystem
      settings: PortSchema="{\"entries\":[{\"content\":{\"sides\":[{\"content\":{\"connectorIds\":[\"In1\",\"In2\"]},\"type\":\"ConnectorPlacement.EquallySpacedRectSide\",\"uuid\":\"b10cca13-b0c2-430a-b17c-db71eb4f1a3c\"},{\"content\":{\"connectorIds\":[\"Out1\",\"Out2\",\"Out3\",\"Out4\"],\"side\":\"RIGHT\"},\"type\":\"ConnectorPlacement.EquallySpacedRectSide\",\"uuid\":\"355382eb-bc30-4f3c-94e5-48c8b9c2ecfd\"},{\"content\":{\"connectorIds\":[\"Out5\",\"Out6\"],\"side\":\"TOP\"},\"type\":\"ConnectorPlacement.EquallySpacedRectSide\",\"uuid\":\"77f94122-ff4d-41eb-b55d-9b38525f3ab4\"}]},\"type\":\"ConnectorPlacement.EquallySpacedConnector\",\"uuid\":\"46538cda-22c7-46a2-9cc9-63f6dc7214f2\"}],\"packageUris\":[\"http://schema.mathworks.com/mf0/Connector/R2020b\"],\"version\":\"1.0\"}"
  Rate Transition{,1..2,7} (4 alike) : RateTransition  OutPortSampleTime=Ts_Control
  Rate Transition11 : RateTransition  OutPortSampleTime=Ts_Power
  Rate Transition3 : RateTransition  OutPortSampleTime=Ts_Power
  Rate Transition4 : RateTransition  OutPortSampleTime=Ts_Power
  Reactive Power Regulator : Subsystem
      settings: PortSchema="{\"entries\":[{\"content\":{\"sides\":[{\"content\":{\"connectorIds\":[\"In1\",\"In2\"]},\"type\":\"ConnectorPlacement.EquallySpacedRectSide\",\"uuid\":\"eeeb811d-908b-486e-b0fa-0b5fd0d6695a\"},{\"content\":{\"connectorIds\":[\"Out1\"],\"side\":\"RIGHT\"},\"type\":\"ConnectorPlacement.EquallySpacedRectSide\",\"uuid\":\"28c9bf02-c5ab-433a-87a9-c17e67d0c029\"},{\"content\":{\"side\":\"TOP\"},\"type\":\"ConnectorPlacement.EquallySpacedRectSide\",\"uuid\":\"fdca837a-4079-4910-a6d7-edbb284eaa51\"},{\"content\":{\"connectorIds\":[\"In3\",\"In4\"],\"side\":\"BOTTOM\"},\"type\":\"ConnectorPlacement.EquallySpacedRectSide\",\"uuid\":\"d2fa5805-110b-4a78-bf6e-301fd334a724\"}]},\"type\":\"ConnectorPlacement.EquallySpacedConnector\",\"uuid\":\"cbc8ea8f-55f5-4ff6-b34f-d5812b415dcf\"}],\"packageUris\":[\"http://schema.mathworks.com/mf0/Connector/R2020b\"],\"version\":\"1.0\"}"
  Switch : Switch  Criteria=u2 ~= 0  SaturateOnIntegerOverflow=off  InputSameDT=off
  Uref : Outport
  Meas : Outport  Port=2
  m1_dq : Outport  Port=3
  wt : Outport  Port=4
  wires:
  Mux1/1 -> Bus Creator/7  "PrefPmeas"
  "PLL, Measurements and Transformation"/4(P) -> Mux1/2, Active Power Regulator (Preg)/1(Pmeas)
  DC Voltage Regulator (VDCreg)/1(Id_ref) -> Mux/1
  "PLL, Measurements and Transformation"/2(wt) -> Rate Transition4/1, Current Regulator (Ireg)/4(wt)
  Demux1/1 -> Bus Creator/3  "Id"
  Vsec/1 -> Rate Transition1/1
  "PLL, Measurements and Transformation"/6(VdVq) -> Reactive Power Regulator/4(VdVq_mes), Current Regulator (Ireg)/2(VdVq)
  Mux2/1 -> [QrefQmeas]
  Rate Transition11/1 -> Uref/1
  "PLL, Measurements and Transformation"/5(Q) -> Mux2/2, Reactive Power Regulator/3(Qmes)
  [Pref] -> Active Power Regulator (Preg)/2(Pref), Mux1/1
  Isec/1 -> Rate Transition2/1
  [PQreg_On] -> Active Power Regulator (Preg)/3(On)
  [QrefQmeas] -> Bus Creator/8  "QrefQmeas"
  Current Regulator (Ireg)/2(m) -> Rate Transition3/1, Rate Transition7/1
  Demux3/2 -> Bus Creator/2  "Iqref"
  Rate Transition7/1 -> Bus Creator/5  "m"
  [Vdc_ref_Preg] -> Switch/1
  Demux3/1 -> Bus Creator/1  "Idref"
  Mux/1 -> Demux3/1, Current Regulator (Ireg)/1(IdIq_ref)
  Switch/1 -> DC Voltage Regulator (VDCreg)/1(Vdc_ref)
  Current Regulator (Ireg)/3(PIdq) -> Bus Creator/6  "PIdq"
  [Vdc1] -> Rate Transition/1
  PQreg_ON/1 -> Reactive Power Regulator/1(On), Switch/2
  Rate Transition1/1 -> "PLL, Measurements and Transformation"/1(Vabc)
  "PLL, Measurements and Transformation"/1(Freq) -> Current Regulator (Ireg)/3(Freq)
  Vdc_ref/1 -> Switch/3
  Active Power Regulator (Preg)/1(Vdc_ref) -> [Vdc_ref_Preg]
  Rate Transition2/1 -> "PLL, Measurements and Transformation"/2(Iabc)
  Rate Transition/1 -> DC Voltage Regulator (VDCreg)/3(Vdc_meas), Current Regulator (Ireg)/6(Vdc)
  [VDCreg_On] -> DC Voltage Regulator (VDCreg)/2(On)
  Demux1/2 -> Bus Creator/4  "Iq"
  "PLL, Measurements and Transformation"/3(IdIq) -> Current Regulator (Ireg)/5(IdIq), Demux1/1
  Qref/1 -> Mux2/1, Reactive Power Regulator/2(Qref)
  Current Regulator (Ireg)/1(Uref_ABC) -> Rate Transition11/1
  Bus Creator/1 -> Meas/1
  Reactive Power Regulator/1(Iq_ref) -> Mux/2
  Rate Transition3/1 -> m1_dq/1
  Rate Transition4/1 -> wt/1
